simulink model "FSK"  (R2021a)
settings: Solver=VariableStepAuto  StartTime=0.0  StopTime=10.0  RelTol=1e-3
libraries: commrandsrc3 x1, commsynccomp2 x1
settings Model: Creator=Dell  LastModifiedBy=Dell

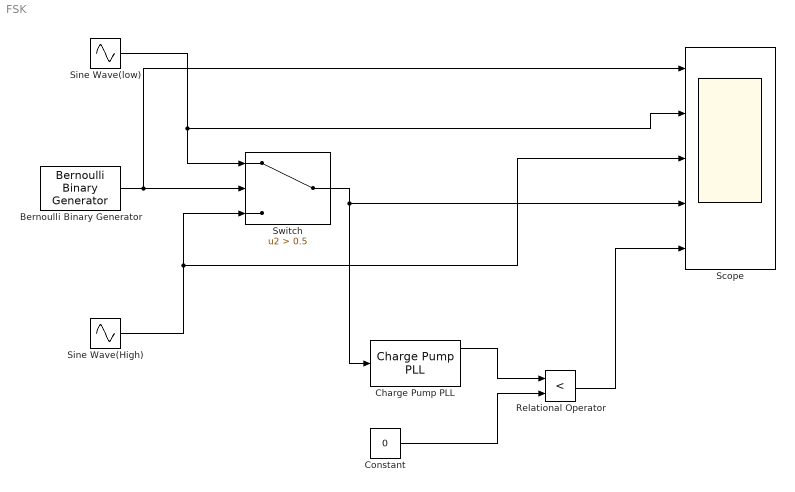
== system FSK ==
  Bernoulli Binary Generator : commrandsrc3/Bernoulli Binary Generator  ProbabilityOfZero=0.5  SeedSource=Auto  Seed=0  SampleTime=1  SamplesPerFrame=1  OutputDataType=double  SimulateUsing=Interpreted execution
  Charge Pump PLL : commsynccomp2/Charge Pump PLL  Fn=[2*pi*1]  Fd="[1  2*pi*1]"  Kvco=4  Fc=10  Ph=0  Ac=1
      settings: SourceProductBaseCode=CM
  Constant : Constant  Value=0
  Relational Operator : RelationalOperator  Operator=<  OutDataTypeStr=boolean  RndMeth=Simplest
  Scope : Scope  NumInputPorts=5
  Sine Wave(High) : Sin  Frequency=2*pi*12  SampleTime=0.01
  Sine Wave(low) : Sin  Frequency=2*pi*4  SampleTime=0.01
  Switch : Switch  Criteria=u2 > Threshold  Threshold=0.5
  wires:
  Sine Wave(low)/1 -> Switch/1, Scope/2
  Sine Wave(High)/1 -> Scope/3, Switch/3
  Bernoulli Binary Generator/1 -> Scope/1, Switch/2
  Switch/1 -> Charge Pump PLL/1, Scope/4
  Charge Pump PLL/1 -> Relational Operator/1
  Constant/1 -> Relational Operator/2
  Relational Operator/1 -> Scope/5
